simulink model "feedback_harness"  (R2013a)
settings: Solver=ode45  StartTime=0.0  StopTime=20  RelTol=1e-3
settings Model: ModifiedByFormat=The MathWorks Inc.  Creator=The MathWorks Inc.  LastModifiedBy=The MathWorks Inc.
settings DataIOCC: SaveOutput=off  SaveTime=off
settings OptimizationCC: ExpressionDepthLimit=2147483647  LifeSpan=1
settings DebuggingCC: FcnCallInpInsideContextMsg=EnableAllAsWarning
settings GRTTargetCC: CombineOutputUpdateFcns=off  GRTInterface=on

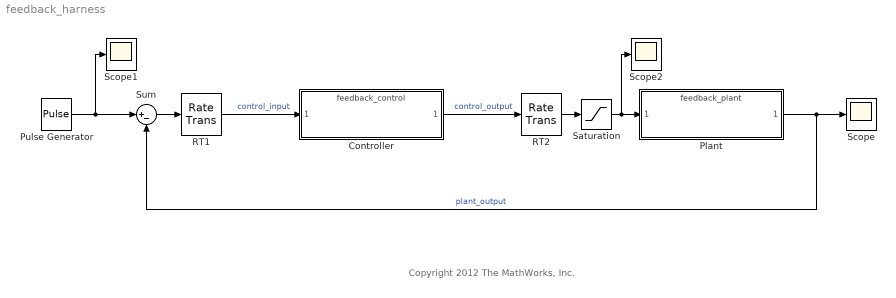
== system feedback_harness ==
  note: Copyright 2012 The MathWorks, Inc.
  Controller : ModelReference  ModelNameDialog=feedback_control  SimulationMode=Normal  ModelReferenceVersion=1.43  CopyOfModelName=feedback_control  DefaultDataLogging=on
  Plant : ModelReference  ModelNameDialog=feedback_plant  SimulationMode=Normal  ModelReferenceVersion=1.23  CopyOfModelName=feedback_plant  DefaultDataLogging=on
  Pulse Generator : DiscretePulseGenerator  PulseType=Time based  Period=4  PulseWidth=50
  RT1 : RateTransition
  RT2 : RateTransition
  Saturation : Saturate  UpperLimit=10  LowerLimit=-10
  Scope : Scope
      settings: TimeRange=1  YMin=0  YMax=1.4
  Scope1 : Scope
  Scope2 : Scope
      settings: SaveName=ScopeData2
  Sum : Sum  Inputs=|+-
  wires:
  Pulse Generator/1 -> Scope1/1, Sum/1
  Sum/1 -> RT1/1
  Controller/1 -> RT2/1  "control_output"
  Plant/1 -> Scope/1, Sum/2  "plant_output"
  RT1/1 -> Controller/1  "control_input"
  RT2/1 -> Saturation/1
  Saturation/1 -> Scope2/1, Plant/1
